simulink model "TaskServiceBase_FSM"  (R2015b)
settings: Solver=ode4  StartTime=0.0  StopTime=inf  FixedStep=.01  RelTol=1e-3
settings Model: Creator=elliocm  LastModifiedBy=elliocm

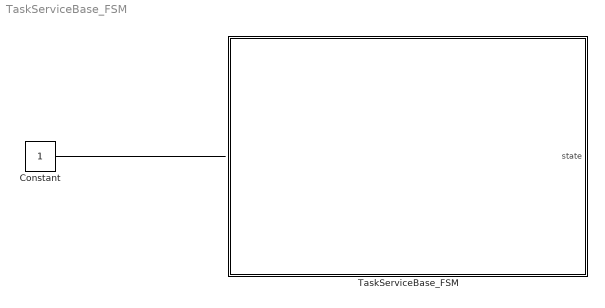
== system TaskServiceBase_FSM ==
  Constant : Constant
  TaskServiceBase_FSM : Stateflow chart  RequirementInfo="{}  %GIDa_69d87331_3a4c_4800_b6a9_49c4bb62fd68"  TreatAsAtomicUnit=on
  wires:
  Constant/1 -> ?

== stateflow chart TaskServiceBase_FSM/TaskServiceBase_FSM ==
  state Idle
    entry: state = 2
    state Init_Request
      entry: UniqueAutomationRequest_in = 0
      unique_automation_request_task_id_present = 0
    note: Simple Delay
        | (Consider Random Fail on TaskInit)
    state Init_Success
      entry: UniqueAutomationRequest_in = 1
      unique_automation_request_task_id_present = 1
    (default) -> Idle.Init_Request
    Idle.Init_Request -> (junction 51)
    (junction 51) -> Idle.Init_Success : after(15,sec)
  state Init
    entry: state = 1
    note: Simple Delay
        | (Consider Random Fail on TaskInit)
    state Init_Request
      entry: init_complete = 0
      TaskInitialized_out = 0
    state Init_Success
      entry: init_complete = 1
      TaskInitialized_out = 1
    (default) -> Init.Init_Request
    Init.Init_Request -> (junction 40)
    (junction 40) -> Init.Init_Success : after(15,sec)
  state SensorRequest
    entry: state = 3
  state OptionRoutes
    entry: state = 4
  state Completed
    entry: state = 9
  state Active
    entry: state = 8
  state OptionSelected
    entry: state = 7
  state OptionsPublished
    entry: state = 5
  state FinalRoutes
    entry: state = 6
  Init -> Idle : [init_complete && TaskInitialized_out]
  (default) -> Init
  Idle -> SensorRequest : [UniqueAutomationRequest_in && unique_automation_request_task_id_present]
  OptionSelected -> SensorRequest [order 1]
  SensorRequest -> OptionRoutes
  Completed -> Idle
  OptionRoutes -> OptionsPublished
  Active -> Completed
  OptionSelected -> Active [order 2]
  OptionsPublished -> FinalRoutes
  FinalRoutes -> OptionSelected
  data: state output; init_complete local; i local; TaskInitialized_out local; UniqueAutomationRequest_in local; unique_automation_request_task_id_present local
